simulink model "Simulink_ControllerARMAX_BlaneRev"  (R2020b)
settings: Solver=VariableStepAuto  StartTime=0.0  StopTime=2400  RelTol=1e-3
values from neighbouring files (symbols this model uses):
  A = [a2, a1, a0]    [Controller_ARMAX_BlaneRev.m]    (also in Controller_SS_BlaneRev.m; Controller_TF_BlaneRev.m = [a1, a0])
  B = [b2, b1, b0]    [Controller_ARMAX_BlaneRev.m]    (also in Controller_SS_BlaneRev.m; Controller_TF_BlaneRev.m = [b1, b0])
  b = double(sol.b)    [Controller_ARMAX_BlaneRev.m]    (also in Controller_SS_BlaneRev.m; Controller_TF_BlaneRev.m = double(sol))
  b_tun = 1    [Controller_ARMAX_BlaneRev.m]    (also in Controller_SS_BlaneRev.m = 0.04062; Controller_TF_BlaneRev.m = 0.008893)
  c = double(sol.c)    [Controller_ARMAX_BlaneRev.m]    (also in Controller_SS_BlaneRev.m)
  c0_Gc = (S0 + S1 + S2)/(1+r0)    [Controller_ARMAX_BlaneRev.m]    (also in Controller_SS_BlaneRev.m)
  c0_Gff = (T_S2 + T_S1 + T_S0)/(1+r0)    [Controller_ARMAX_BlaneRev.m]    (also in Controller_SS_BlaneRev.m)
  c_tun = 1    [Controller_ARMAX_BlaneRev.m]    (also in Controller_SS_BlaneRev.m = 0.0007977)
  D = double(sol.D)    [Controller_ARMAX_BlaneRev.m]    (also in Controller_SS_BlaneRev.m)
  D_tun = 109.2    [Controller_ARMAX_BlaneRev.m]    (also in Controller_SS_BlaneRev.m = 126.3)
  Gp = tf(sysARMAX)    [Controller_ARMAX_BlaneRev.m]    (also in Controller_SS_BlaneRev.m = tf(B, A, Ts2); Controller_TF_BlaneRev.m = tf(sysTF))
  Gp_cont = d2c(Gp_origin, 'zoh')    [Controller_ARMAX_BlaneRev.m]    (also in Controller_SS_BlaneRev.m; Controller_TF_BlaneRev.m = d2c(Gp, 'zoh'))
  I = double(sol.I)    [Controller_ARMAX_BlaneRev.m]    (also in Controller_SS_BlaneRev.m; Controller_TF_BlaneRev.m)
  I_tun = .06907    (= 0.06907)    [Controller_ARMAX_BlaneRev.m]    (also in Controller_SS_BlaneRev.m = 0.1006; Controller_TF_BlaneRev.m = 0.08704)
  N = double(sol.N)    [Controller_ARMAX_BlaneRev.m]    (also in Controller_SS_BlaneRev.m; systemIdentification_47414_Blane.m = 5; systemIdentification_48404_Blane.m = 5; systemIdentification_49404_Blane.m = 5)
  N_tun = .6217    (= 0.6217)    [Controller_ARMAX_BlaneRev.m]    (also in Controller_SS_BlaneRev.m = 0.5253)
  P = double(sol.P)    [Controller_ARMAX_BlaneRev.m]    (also in Controller_SS_BlaneRev.m; Controller_TF_BlaneRev.m)
  P_tun = 5.628    [Controller_ARMAX_BlaneRev.m]    (also in Controller_SS_BlaneRev.m = 7.185; Controller_TF_BlaneRev.m = 3.173)
  PD_den = [1, r0]    [Controller_ARMAX_BlaneRev.m]    (also in Controller_SS_BlaneRev.m)
  PD_SR_num = [d1_Gc, d0_Gc]    [Controller_ARMAX_BlaneRev.m]    (also in Controller_SS_BlaneRev.m)
  PD_TR_num = [d1_Gff, d0_Gff]    [Controller_ARMAX_BlaneRev.m]    (also in Controller_SS_BlaneRev.m)
  Ts = .4    (= 0.4)    [Controller_ARMAX_BlaneRev.m]    (also in Controller_SS_BlaneRev.m; Controller_TF_BlaneRev.m; systemIdentification_47414_Blane.m = 0.2; systemIdentification_48404_Blane.m = 1)
  Ts2 = .4    (= 0.4)    [Controller_ARMAX_BlaneRev.m]    (also in Controller_SS_BlaneRev.m; Controller_TF_BlaneRev.m)
  Ts3 = 1    [Controller_ARMAX_BlaneRev.m]    (also in Controller_SS_BlaneRev.m; Controller_TF_BlaneRev.m)
undefined symbols (not defined in the file or in its folder): DiscIntNeverNeededParam, K_ant
libraries: simulink_extras x8, pid_lib x2
settings Model: Creator=Blane Brinkley  LastModifiedBy=Blane Brinkley

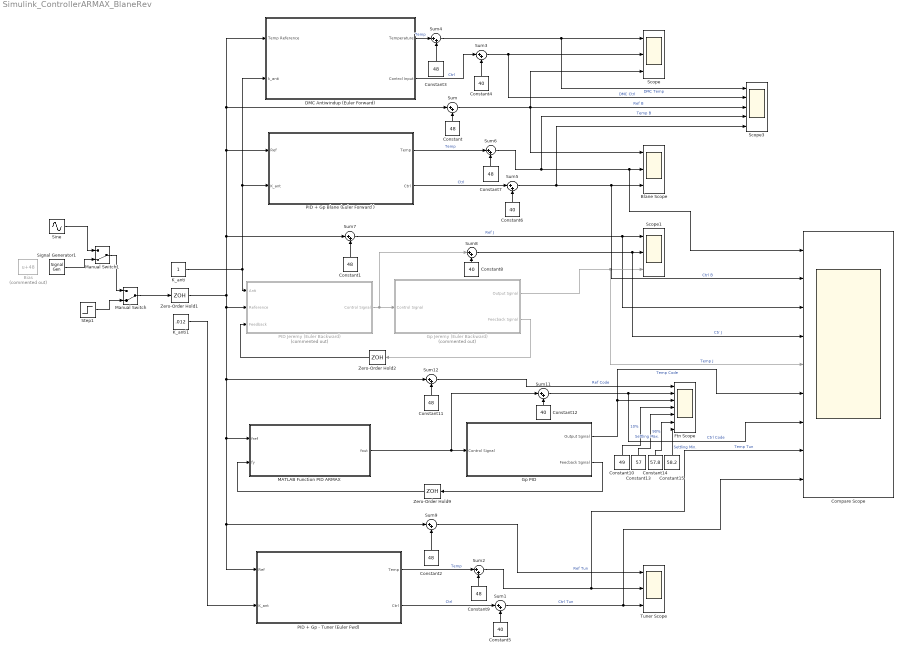
== system Simulink_ControllerARMAX_BlaneRev ==
  Bias : Bias  Commented=on  Bias=48
  Blane Scope : Scope  NumInputPorts=3
  Compare Scope : Scope  NumInputPorts=9
  Constant{,1..3,7,9,11} (7 alike) : Constant  Value=48
  Constant10 : Constant  Value=49
  Constant{4..6,8,12} (5 alike) : Constant  Value=40
  Constant13 : Constant  Value=57
  Constant14 : Constant  Value=57.8
  Constant15 : Constant  Value=58.2
  DMC Antiwindup (Euler Forward) : Subsystem
  Ftn Scope : Scope  NumInputPorts=7
  Gp Jeremy (Euler Backward) : Subsystem  Commented=on
  "Gp PID " : Subsystem
  K_anti : Constant
  K_anti1 : Constant  Value=.012  VectorParams1D=off
  MATLAB Function PID ARMAX : MATLAB Function  TreatAsAtomicUnit=on
  Manual Switch : ManualSwitch  CurrentSetting=0
  Manual Switch1 : ManualSwitch  CurrentSetting=0
  PID + Gp - Tuner (Euler Fwd) : Subsystem
  PID + Gp Blane (Euler Forward ) : Subsystem
  PID Jeremy (Euler Backward) : Subsystem  Commented=on
  Scope : Scope  NumInputPorts=3
  Scope1 : Scope  NumInputPorts=3
  Scope3 : Scope  NumInputPorts=5
  Signal Generator1 : SignalGenerator  WaveForm=square  Amplitude=20  Frequency=1/1200
  Sine : Sin  Amplitude=10  Frequency=1/1200*6.28  SampleTime=0
  Step1 : Step  Time=0  After=10  SampleTime=Ts
  Sum{,1..9,11..12} (12 alike) : Sum  Inputs=|++
  Tuner Scope : Scope  NumInputPorts=3
  Zero-Order Hold1 : ZeroOrderHold  SampleTime=Ts3
  Zero-Order Hold2 : ZeroOrderHold  SampleTime=Ts3
  Zero-Order Hold9 : ZeroOrderHold  SampleTime=Ts3
  wires:
  Signal Generator1/1 -> Manual Switch1/2
  Constant15/1 -> Ftn Scope/7  "Settling Min."
  Sine/1 -> Manual Switch1/1
  Manual Switch1/1 -> Manual Switch/1
  Constant14/1 -> Ftn Scope/6  "Settling Max."
  Step1/1 -> Manual Switch/2
  Zero-Order Hold2/1 -> PID Jeremy (Euler Backward)/3(Feedback)
  Constant2/1 -> Sum9/2
  Sum12/1 -> Ftn Scope/1  "Ref Code"
  Sum7/1 -> Compare Scope/3, Scope1/1  "Ref J"
  Constant3/1 -> Sum4/2
  Constant7/1 -> Sum6/2
  Constant4/1 -> Sum3/2
  PID Jeremy (Euler Backward)/1(Control Signal) -> Sum8/1, Gp Jeremy (Euler Backward)/1(Control Signal)
  Zero-Order Hold1/1 -> PID Jeremy (Euler Backward)/2(Reference), Sum12/1, PID + Gp - Tuner (Euler Fwd)/1(Ref), Sum9/1, MATLAB Function PID ARMAX/1(fref), DMC Antiwindup (Euler Forward)/1(Temp Reference), Sum/1, PID + Gp Blane (Euler Forward )/1(Ref), Sum7/1
  Sum/1 -> Scope3/3, Scope/3, Blane Scope/1  "Ref B"
  Sum4/1 -> Scope/1, Scope3/1  "DMC Temp"
  Constant/1 -> Sum/2
  DMC Antiwindup (Euler Forward)/1("Temperature ") -> Sum4/1  "Temp"
  Sum6/1 -> Scope3/4, Compare Scope/1, Blane Scope/2  "Temp B"
  PID + Gp Blane (Euler Forward )/1(Temp) -> Sum6/1  "Temp"
  Constant6/1 -> Sum5/2
  Constant1/1 -> Sum7/2
  Sum2/1 -> Compare Scope/8, Tuner Scope/2  "Temp Tun"
  Manual Switch/1 -> Zero-Order Hold1/1
  PID + Gp Blane (Euler Forward )/2(Ctrl) -> Sum5/1  "Ctrl"
  MATLAB Function PID ARMAX/1(fout) -> Sum11/1, "Gp PID "/1(Control Signal)
  "Gp PID "/1(Output Sginal) -> Compare Scope/6, Ftn Scope/3  "Temp Code"
  Gp Jeremy (Euler Backward)/1(Output Sginal) -> Compare Scope/5, Scope1/3  "Temp J"
  Sum5/1 -> Scope3/5, Compare Scope/2, Blane Scope/3  "Ctrl B"
  Sum8/1 -> Compare Scope/4, Scope1/2  "Ctr J"
  Constant12/1 -> Sum11/2
  DMC Antiwindup (Euler Forward)/2("Control Input ") -> Sum3/1  "Ctrl"
  Constant8/1 -> Sum8/2
  K_anti1/1 -> PID + Gp - Tuner (Euler Fwd)/2(K_ant)
  PID + Gp - Tuner (Euler Fwd)/2(Ctrl) -> Sum1/1  "Ctrl"
  Sum11/1 -> Compare Scope/7, Ftn Scope/2  "Ctrl Code"
  Sum1/1 -> Tuner Scope/3, Compare Scope/9  "Ctrl Tun"
  K_anti/1 -> PID Jeremy (Euler Backward)/1(Anti), DMC Antiwindup (Euler Forward)/2(k_anti), PID + Gp Blane (Euler Forward )/2(K_ant)
  "Gp PID "/2(Feecback Sginal) -> Zero-Order Hold9/1
  Constant9/1 -> Sum2/2
  Sum9/1 -> Tuner Scope/1  "Ref Tun"
  Constant5/1 -> Sum1/2
  Sum3/1 -> Scope/2, Scope3/2  "DMC Ctrl"
  Constant11/1 -> Sum12/2
  Gp Jeremy (Euler Backward)/2(Feecback Sginal) -> Zero-Order Hold2/1
  Zero-Order Hold9/1 -> MATLAB Function PID ARMAX/2(fy)
  Constant10/1 -> Ftn Scope/4  "10%"
  PID + Gp - Tuner (Euler Fwd)/1(Temp) -> Sum2/1  "Temp"
  Constant13/1 -> Ftn Scope/5  "90%"

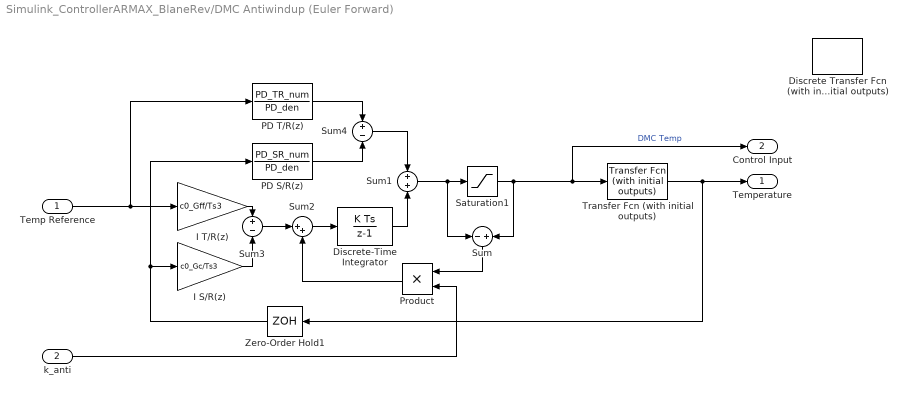
== system Simulink_ControllerARMAX_BlaneRev/DMC Antiwindup (Euler Forward) ==
  Temp Reference : Inport
  k_anti : Inport  Port=2
  Discrete Transfer Fcn (with initial outputs) : simulink_extras/Additional Discrete/Discrete Transfer Fcn (with initial outputs)  N=Gp.Numerator{1}  D=Gp.Denominator{1}  U0=[1]  Y0=0  TS=Ts
      settings: SourceProductBaseCode=SL
  Discrete-Time Integrator : DiscreteIntegrator  SampleTime=Ts3  ICPrevOutput=DiscIntNeverNeededParam  ICPrevScaledInput=DiscIntNeverNeededParam
  I S/R(z) : Gain  Gain=c0_Gc/Ts3
  I T/R(z) : Gain  Gain=c0_Gff/Ts3
  PD S/R(z) : DiscreteTransferFcn  Numerator=PD_SR_num  Denominator=PD_den  SampleTime=Ts3
  PD T/R(z) : DiscreteTransferFcn  Numerator=PD_TR_num  Denominator=PD_den  SampleTime=Ts3
  Product : Product
  Saturation1 : Saturate  UpperLimit=60  LowerLimit=-40
  Sum : Sum  Inputs=-+
  Sum1 : Sum
  Sum2 : Sum  Inputs=|++
  Sum3 : Sum  Inputs=+-
  Sum4 : Sum  Inputs=+-
  Transfer Fcn (with initial outputs) : simulink_extras/Additional Linear/Transfer Fcn (with initial outputs)  N=Gp_cont.Numerator{1}  D=Gp_cont.Denominator{1}  Y0=0  U0=0
  Zero-Order Hold1 : ZeroOrderHold  SampleTime=Ts3
  "Temperature " : Outport
  "Control Input " : Outport  Port=2
  wires:
  Sum3/1 -> Sum2/1
  I S/R(z)/1 -> Sum3/2
  Sum2/1 -> Discrete-Time Integrator/1
  I T/R(z)/1 -> Sum3/1
  Discrete-Time Integrator/1 -> Sum1/2
  Sum1/1 -> Sum/1, Saturation1/1
  Sum/1 -> Product/1
  Sum4/1 -> Sum1/1
  PD S/R(z)/1 -> Sum4/2
  PD T/R(z)/1 -> Sum4/1
  Product/1 -> Sum2/2
  Temp Reference/1 -> PD T/R(z)/1, I T/R(z)/1
  Transfer Fcn (with initial outputs)/1 -> Zero-Order Hold1/1, "Temperature "/1
  Zero-Order Hold1/1 -> I S/R(z)/1, PD S/R(z)/1
  Saturation1/1 -> Transfer Fcn (with initial outputs)/1, "Control Input "/1, Sum/2  "DMC Temp"
  k_anti/1 -> Product/2

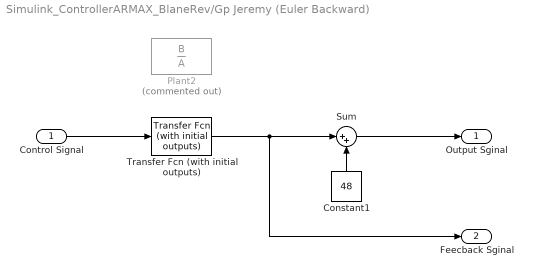
== system Simulink_ControllerARMAX_BlaneRev/Gp Jeremy (Euler Backward) ==
  Control Signal : Inport
  Constant1 : Constant  Value=48
  Plant2 : DiscreteTransferFcn  Commented=on  Numerator=B  Denominator=A  SampleTime=0.4
  Sum : Sum  Inputs=|++
  Transfer Fcn (with initial outputs) : simulink_extras/Additional Linear/Transfer Fcn (with initial outputs)  N=Gp_cont.Numerator{1}  D=Gp_cont.Denominator{1}  Y0=0  U0=0
  Output Sginal : Outport
  Feecback Sginal : Outport  Port=2
  wires:
  Transfer Fcn (with initial outputs)/1 -> Feecback Sginal/1, Sum/1
  Sum/1 -> Output Sginal/1
  Constant1/1 -> Sum/2
  Control Signal/1 -> Transfer Fcn (with initial outputs)/1

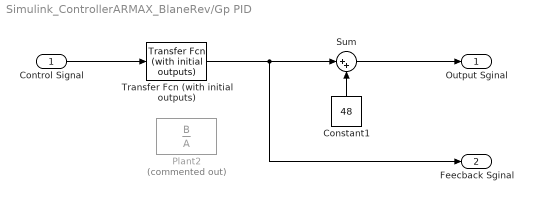
== system Simulink_ControllerARMAX_BlaneRev/Gp PID  ==
  Control Signal : Inport
  Constant1 : Constant  Value=48
  Plant2 : DiscreteTransferFcn  Commented=on  Numerator=B  Denominator=A  SampleTime=0.4
  Sum : Sum  Inputs=|++
  Transfer Fcn (with initial outputs) : simulink_extras/Additional Linear/Transfer Fcn (with initial outputs)  N=Gp_cont.Numerator{1}  D=Gp_cont.Denominator{1}  Y0=0  U0=0
  Output Sginal : Outport
  Feecback Sginal : Outport  Port=2
  wires:
  Transfer Fcn (with initial outputs)/1 -> Feecback Sginal/1, Sum/1
  Sum/1 -> Output Sginal/1
  Constant1/1 -> Sum/2
  Control Signal/1 -> Transfer Fcn (with initial outputs)/1

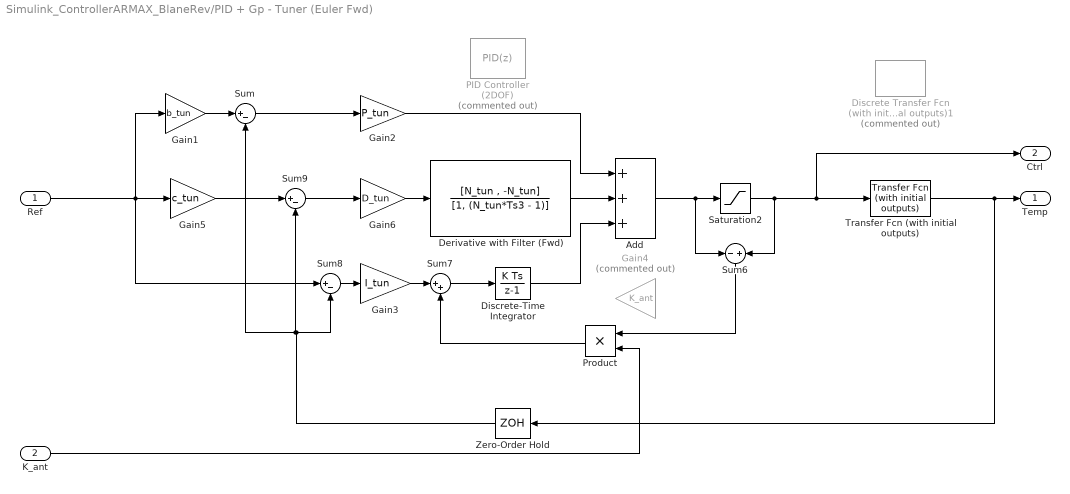
== system Simulink_ControllerARMAX_BlaneRev/PID + Gp - Tuner (Euler Fwd) ==
  Ref : Inport
  K_ant : Inport  Port=2
  Add : Sum  Inputs=+++
  Derivative with Filter (Fwd) : DiscreteTransferFcn  Numerator=[N_tun , -N_tun]  Denominator=[1, (N_tun*Ts3 - 1)]  SampleTime=Ts3
  Discrete Transfer Fcn (with initial outputs)1 : simulink_extras/Additional Discrete/Discrete Transfer Fcn (with initial outputs)  Commented=on  N=Gp.Numerator{1}  D=Gp.Denominator{1}  U0=[1]  Y0=0  TS=Ts
      settings: SourceProductBaseCode=SL
  Discrete-Time Integrator : DiscreteIntegrator  SampleTime=Ts3  ICPrevOutput=DiscIntNeverNeededParam  ICPrevScaledInput=DiscIntNeverNeededParam
  Gain1 : Gain  Gain=b_tun
  Gain2 : Gain  Gain=P_tun
  Gain3 : Gain  Gain=I_tun
  Gain4 : Gain  Commented=on  Gain=K_ant
  Gain5 : Gain  Gain=c_tun
  Gain6 : Gain  Gain=D_tun
  PID Controller (2DOF) : pid_lib/PID Controller (2DOF)  Commented=on  Controller=PID  Form=Parallel  TimeDomain=Discrete-time  UseExternalTs=off  SampleTime=-1  IntegratorMethod=Forward Euler  FilterMethod=Forward Euler  ControllerParametersSource=internal  P=1  I=1  D=0  UseFilter=on  N=100  b=1  c=1  TunerSelectOption=Transfer Function Based (PID Tuner App)  InitialConditionSource=internal  InitialConditionForIntegrator=0  InitialConditionForFilter=0  DifferentiatorICPrevScaledInput=0  ExternalReset=none  TrackingMode=off  Kt=1  LimitOutput=off  SatLimitsSource=internal  UpperSaturationLimit=inf  LowerSaturationLimit=-inf  LinearizeAsGain=on  AntiWindupMode=none  Kb=1  POutMin=[]  POutMax=[]  IOutMin=[]  IOutMax=[]  DOutMin=[]  DOutMax=[]  NOutMin=[]  NOutMax=[]  bOutMin=[]  bOutMax=[]  cOutMin=[]  cOutMax=[]  SumOutMin=[]  SumOutMax=[]  SaturationOutMin=[]  SaturationOutMax=[]  PParamMin=[]  PParamMax=[]  IParamMin=[]  IParamMax=[]  DParamMin=[]  DParamMax=[]  NParamMin=[]  NParamMax=[]  bParamMin=[]  bParamMax=[]  cParamMin=[]  cParamMax=[]  KbParamMin=[]  KbParamMax=[]  KtParamMin=[]  KtParamMax=[]  KbOutMin=[]  KbOutMax=[]  KtOutMin=[]  KtOutMax=[]  IntegratorOutMin=[]  IntegratorOutMax=[]  FilterOutMin=[]  FilterOutMax=[]  SumI1OutMin=[]  SumI1OutMax=[]  SumI2OutMin=[]  SumI2OutMax=[]  SumI3OutMin=[]  SumI3OutMax=[]  SumI4OutMin=[]  SumI4OutMax=[]  SumDOutMin=[]  SumDOutMax=[]  Sum1OutMin=[]  Sum1OutMax=[]  Sum2OutMin=[]  Sum2OutMax=[]  Sum3OutMin=[]  Sum3OutMax=[]  DifferentiatorOutMin=[]  DifferentiatorOutMax=[]  FilterDiffOutCoefMin=[]  FilterDiffOutCoefMax=[]  ReciprocalOutMin=[]  ReciprocalOutMax=[]  SumDenOutMin=[]  SumDenOutMax=[]  SumNumOutMin=[]  SumNumOutMax=[]  DivideOutMin=[]  DivideOutMax=[]  UdiffTsProdOutMin=[]  UdiffTsProdOutMax=[]  NTsProdOutMin=[]  NTsProdOutMax=[]  UintegralTsProdOutMin=[]  UintegralTsProdOutMax=[]  UngainTsProdOutMin=[]  UngainTsProdOutMax=[]  IntegratorContinuousStateAttributes=''  IntegratorStateMustResolveToSignalObject=off  IntegratorRTWStateStorageClass=Auto  FilterContinuousStateAttributes=''  FilterStateMustResolveToSignalObject=off  FilterRTWStateStorageClass=Auto  ParallelPVariant=InternalParameters  IdealPVariant=Disabled  IVariant=InternalParameters  DVariant=InternalParameters  bVariant=InternalParameters  cVariant=InternalParameters  IntegratorVariant=Discrete  SatVariant=Disabled  AWVariant=Passthrough  PCopyVariant=Disabled  TRVariant=Disabled  FdbkBlocksVariant=Forward  IdealPFdbkVariant=Disabled  SatFdbkVariant=Disabled  DerivativeFilterVariant=ForwardEulerFilter  NVariant=InternalParameters  NCopyVariant=Disabled  FilterICVariant=InternalICsFilter  IntegratorICVariant=InternalICs  ExternalResetVariant=Disabled  TRSumVariant=Passthrough  SumFdbkVariant=Disabled  SumVariant=Sum_PID  TsampFilterVariant=InternalTs  TsampNgainVariant=Passthrough  TsampIntegralVariant=Passthrough  ExternalSaturationOutDataTypeStr=Inherit: Same as second input
      settings: SourceProductBaseCode=SL
  Product : Product
  Saturation2 : Saturate  UpperLimit=60  LowerLimit=-40
  Sum : Sum  Inputs=|+-
  Sum6 : Sum  Inputs=-+
  Sum7 : Sum  Inputs=|++
  Sum8 : Sum  Inputs=|+-
  Sum9 : Sum  Inputs=|+-
  Transfer Fcn (with initial outputs) : simulink_extras/Additional Linear/Transfer Fcn (with initial outputs)  N=Gp_cont.Numerator{1}  D=Gp_cont.Denominator{1}  Y0=0  U0=0
  Zero-Order Hold : ZeroOrderHold  SampleTime=Ts3
  Temp : Outport
  Ctrl : Outport  Port=2
  wires:
  Gain1/1 -> Sum/1
  Sum/1 -> Gain2/1
  Sum8/1 -> Gain3/1
  Sum6/1 -> Product/1
  Add/1 -> Sum6/1, Saturation2/1
  Sum7/1 -> Discrete-Time Integrator/1
  Transfer Fcn (with initial outputs)/1 -> Zero-Order Hold/1, Temp/1
  Gain5/1 -> Sum9/1
  Sum9/1 -> Gain6/1
  Gain2/1 -> Add/1
  Gain6/1 -> Derivative with Filter (Fwd)/1
  Derivative with Filter (Fwd)/1 -> Add/2
  Product/1 -> Sum7/2
  Discrete-Time Integrator/1 -> Add/3
  Gain3/1 -> Sum7/1
  Saturation2/1 -> Sum6/2, Transfer Fcn (with initial outputs)/1, Ctrl/1
  Zero-Order Hold/1 -> Sum8/2, Sum9/2, Sum/2
  Ref/1 -> Sum8/1, Gain5/1, Gain1/1
  K_ant/1 -> Product/2

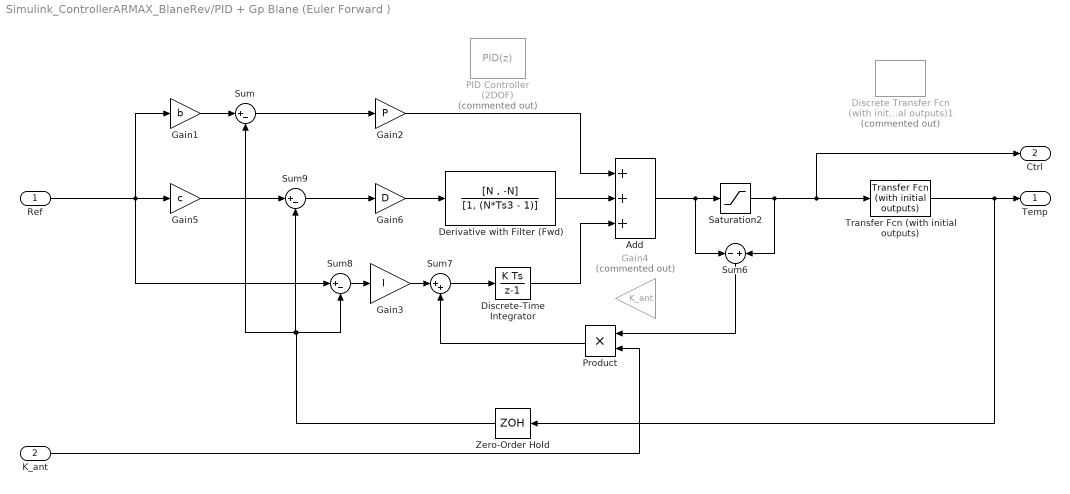
== system Simulink_ControllerARMAX_BlaneRev/PID + Gp Blane (Euler Forward ) ==
  Ref : Inport
  K_ant : Inport  Port=2
  Add : Sum  Inputs=+++
  Derivative with Filter (Fwd) : DiscreteTransferFcn  Numerator=[N , -N]  Denominator=[1, (N*Ts3 - 1)]  SampleTime=Ts3
  Discrete Transfer Fcn (with initial outputs)1 : simulink_extras/Additional Discrete/Discrete Transfer Fcn (with initial outputs)  Commented=on  N=Gp.Numerator{1}  D=Gp.Denominator{1}  U0=[1]  Y0=0  TS=Ts
      settings: SourceProductBaseCode=SL
  Discrete-Time Integrator : DiscreteIntegrator  SampleTime=Ts3  ICPrevOutput=DiscIntNeverNeededParam  ICPrevScaledInput=DiscIntNeverNeededParam
  Gain1 : Gain  Gain=b
  Gain2 : Gain  Gain=P
  Gain3 : Gain  Gain=I
  Gain4 : Gain  Commented=on  Gain=K_ant
  Gain5 : Gain  Gain=c
  Gain6 : Gain  Gain=D
  PID Controller (2DOF) : pid_lib/PID Controller (2DOF)  Commented=on  Controller=PID  Form=Parallel  TimeDomain=Discrete-time  UseExternalTs=off  SampleTime=-1  IntegratorMethod=Forward Euler  FilterMethod=Forward Euler  ControllerParametersSource=internal  P=1  I=1  D=0  UseFilter=on  N=100  b=1  c=1  TunerSelectOption=Transfer Function Based (PID Tuner App)  InitialConditionSource=internal  InitialConditionForIntegrator=0  InitialConditionForFilter=0  DifferentiatorICPrevScaledInput=0  ExternalReset=none  TrackingMode=off  Kt=1  LimitOutput=off  SatLimitsSource=internal  UpperSaturationLimit=inf  LowerSaturationLimit=-inf  LinearizeAsGain=on  AntiWindupMode=none  Kb=1  POutMin=[]  POutMax=[]  IOutMin=[]  IOutMax=[]  DOutMin=[]  DOutMax=[]  NOutMin=[]  NOutMax=[]  bOutMin=[]  bOutMax=[]  cOutMin=[]  cOutMax=[]  SumOutMin=[]  SumOutMax=[]  SaturationOutMin=[]  SaturationOutMax=[]  PParamMin=[]  PParamMax=[]  IParamMin=[]  IParamMax=[]  DParamMin=[]  DParamMax=[]  NParamMin=[]  NParamMax=[]  bParamMin=[]  bParamMax=[]  cParamMin=[]  cParamMax=[]  KbParamMin=[]  KbParamMax=[]  KtParamMin=[]  KtParamMax=[]  KbOutMin=[]  KbOutMax=[]  KtOutMin=[]  KtOutMax=[]  IntegratorOutMin=[]  IntegratorOutMax=[]  FilterOutMin=[]  FilterOutMax=[]  SumI1OutMin=[]  SumI1OutMax=[]  SumI2OutMin=[]  SumI2OutMax=[]  SumI3OutMin=[]  SumI3OutMax=[]  SumI4OutMin=[]  SumI4OutMax=[]  SumDOutMin=[]  SumDOutMax=[]  Sum1OutMin=[]  Sum1OutMax=[]  Sum2OutMin=[]  Sum2OutMax=[]  Sum3OutMin=[]  Sum3OutMax=[]  DifferentiatorOutMin=[]  DifferentiatorOutMax=[]  FilterDiffOutCoefMin=[]  FilterDiffOutCoefMax=[]  ReciprocalOutMin=[]  ReciprocalOutMax=[]  SumDenOutMin=[]  SumDenOutMax=[]  SumNumOutMin=[]  SumNumOutMax=[]  DivideOutMin=[]  DivideOutMax=[]  UdiffTsProdOutMin=[]  UdiffTsProdOutMax=[]  NTsProdOutMin=[]  NTsProdOutMax=[]  UintegralTsProdOutMin=[]  UintegralTsProdOutMax=[]  UngainTsProdOutMin=[]  UngainTsProdOutMax=[]  IntegratorContinuousStateAttributes=''  IntegratorStateMustResolveToSignalObject=off  IntegratorRTWStateStorageClass=Auto  FilterContinuousStateAttributes=''  FilterStateMustResolveToSignalObject=off  FilterRTWStateStorageClass=Auto  ParallelPVariant=InternalParameters  IdealPVariant=Disabled  IVariant=InternalParameters  DVariant=InternalParameters  bVariant=InternalParameters  cVariant=InternalParameters  IntegratorVariant=Discrete  SatVariant=Disabled  AWVariant=Passthrough  PCopyVariant=Disabled  TRVariant=Disabled  FdbkBlocksVariant=Forward  IdealPFdbkVariant=Disabled  SatFdbkVariant=Disabled  DerivativeFilterVariant=ForwardEulerFilter  NVariant=InternalParameters  NCopyVariant=Disabled  FilterICVariant=InternalICsFilter  IntegratorICVariant=InternalICs  ExternalResetVariant=Disabled  TRSumVariant=Passthrough  SumFdbkVariant=Disabled  SumVariant=Sum_PID  TsampFilterVariant=InternalTs  TsampNgainVariant=Passthrough  TsampIntegralVariant=Passthrough  ExternalSaturationOutDataTypeStr=Inherit: Same as second input
      settings: SourceProductBaseCode=SL
  Product : Product
  Saturation2 : Saturate  UpperLimit=60  LowerLimit=-40
  Sum : Sum  Inputs=|+-
  Sum6 : Sum  Inputs=-+
  Sum7 : Sum  Inputs=|++
  Sum8 : Sum  Inputs=|+-
  Sum9 : Sum  Inputs=|+-
  Transfer Fcn (with initial outputs) : simulink_extras/Additional Linear/Transfer Fcn (with initial outputs)  N=Gp_cont.Numerator{1}  D=Gp_cont.Denominator{1}  Y0=0  U0=0
  Zero-Order Hold : ZeroOrderHold  SampleTime=Ts3
  Temp : Outport
  Ctrl : Outport  Port=2
  wires:
  Gain1/1 -> Sum/1
  Sum/1 -> Gain2/1
  Sum8/1 -> Gain3/1
  Sum6/1 -> Product/1
  Add/1 -> Sum6/1, Saturation2/1
  Sum7/1 -> Discrete-Time Integrator/1
  Transfer Fcn (with initial outputs)/1 -> Zero-Order Hold/1, Temp/1
  Gain5/1 -> Sum9/1
  Sum9/1 -> Gain6/1
  Gain2/1 -> Add/1
  Gain6/1 -> Derivative with Filter (Fwd)/1
  Derivative with Filter (Fwd)/1 -> Add/2
  Product/1 -> Sum7/2
  Discrete-Time Integrator/1 -> Add/3
  Gain3/1 -> Sum7/1
  Saturation2/1 -> Sum6/2, Transfer Fcn (with initial outputs)/1, Ctrl/1
  Zero-Order Hold/1 -> Sum8/2, Sum9/2, Sum/2
  Ref/1 -> Sum8/1, Gain1/1, Gain5/1
  K_ant/1 -> Product/2

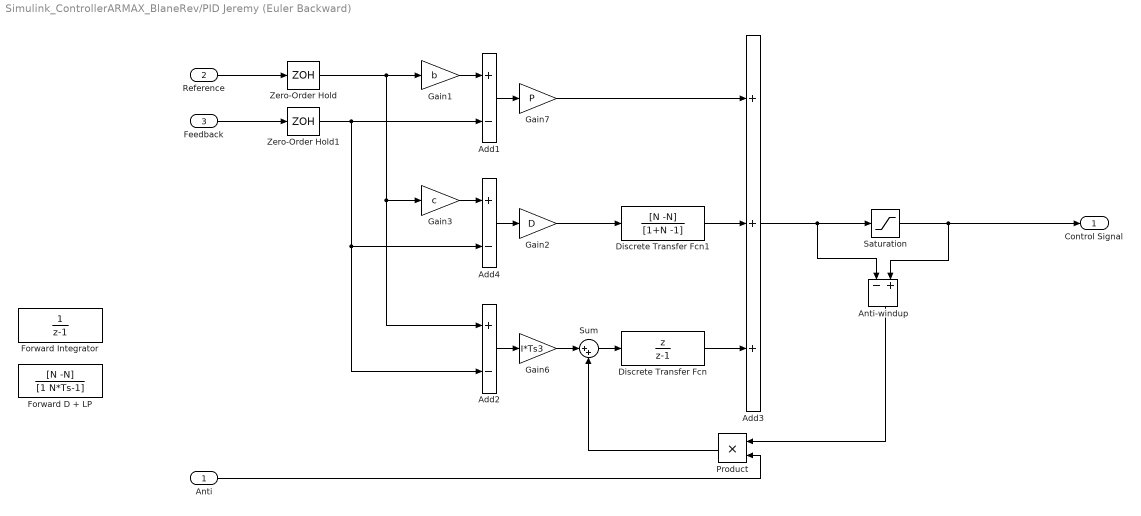
== system Simulink_ControllerARMAX_BlaneRev/PID Jeremy (Euler Backward) ==
  Anti : Inport
  Reference : Inport  Port=2
  Feedback : Inport  Port=3
  Add1 : Sum  Inputs=+-
  Add2 : Sum  Inputs=+-
  Add3 : Sum  Inputs=+++
  Add4 : Sum  Inputs=+-
  Anti-windup : Sum  Inputs=-+
  Discrete Transfer Fcn : DiscreteTransferFcn  Numerator=[1 0]  Denominator=[1 -1]  SampleTime=Ts2
  Discrete Transfer Fcn1 : DiscreteTransferFcn  Numerator=[N -N]  Denominator=[1+N -1]  SampleTime=Ts2
  Forward D + LP : DiscreteTransferFcn  Numerator=[N -N]  Denominator=[1 N*Ts-1]  SampleTime=Ts
  Forward Integrator : DiscreteTransferFcn  Denominator=[1 -1]  SampleTime=Ts
  Gain1 : Gain  Gain=b
  Gain2 : Gain  Gain=D
  Gain3 : Gain  Gain=c
  Gain6 : Gain  Gain=I*Ts3
  Gain7 : Gain  Gain=P
  Product : Product
  Saturation : Saturate  UpperLimit=60  LowerLimit=-40
  Sum : Sum  Inputs=|++
  Zero-Order Hold : ZeroOrderHold  SampleTime=Ts3
  Zero-Order Hold1 : ZeroOrderHold  SampleTime=Ts3
  Control Signal : Outport
  wires:
  Gain1/1 -> Add1/1
  Zero-Order Hold/1 -> Gain1/1, Gain3/1, Add2/1
  Reference/1 -> Zero-Order Hold/1
  Anti-windup/1 -> Product/1
  Product/1 -> Sum/2
  Add3/1 -> Saturation/1, Anti-windup/1
  Gain3/1 -> Add4/1
  Discrete Transfer Fcn1/1 -> Add3/2
  Add1/1 -> Gain7/1
  Gain7/1 -> Add3/1
  Add4/1 -> Gain2/1
  Gain2/1 -> Discrete Transfer Fcn1/1
  Add2/1 -> Gain6/1
  Discrete Transfer Fcn/1 -> Add3/3
  Sum/1 -> Discrete Transfer Fcn/1
  Gain6/1 -> Sum/1
  Feedback/1 -> Zero-Order Hold1/1
  Zero-Order Hold1/1 -> Add1/2, Add4/2, Add2/2
  Saturation/1 -> Control Signal/1, Anti-windup/2
  Anti/1 -> Product/2

== matlab function Simulink_ControllerARMAX_BlaneRev/MATLAB Function PID ARMAX ==
  data: fref input; fout output; fy input
function fout = fcn(fref, fy)
%%%%%%%%%%%%%%%%%%%%%%%%%%%%%%%%%%%%%%%%%%%%%%%%%%%%%%%
% PID + LP + PP for ARMAX
% Input : fref - reference signal
%         fy   - feedback signal
% Output: fout - control signal
%%%%%%%%%%%%%%%%%%%%%%%%%%%%%%%%%%%%%%%%%%%%%%%%%%%%%%%
% Variable Initialisation
persistent fD_prev fI_prev fIA_prev fDErr_prev fant;

% % Blane - SMALL ()
% Ts = 1;
% P = 8.1299;
% I = 0.1071;
% D = 109.7073;
% N = 0.1077;
% b = 0.8236;
% c = 0.6920;
% Kant = .045;

% Jeremy - SMALL ()
Ts = 1;
P = 2.987;
I = .03895;
D = 5.816;
N = .851;
b = 1;
c = 1;
Kant = .12;

% ----------------------------------------

% % Blane - LARGE (60.17 sec)
% Ts = 1;
% P = 57.5573;
% I = 1.5134;
% D = 923.3159;
% N = .5725;
% b = .1292;
% c = .0041;
% Kant = 1;

% % Jeremy - LARGE():
% Ts = 1;
% P = 5.628;
% I = .06907;
% D = 109.2;
% N = .6217;
% b = 1;
% c = 1;
% Kant = .012;

if isempty(fD_prev)
    fD_prev = 0;
    fI_prev = 0;
    fIA_prev = 0;
    fDErr_prev = 0;
    fant = 0;
    
end

fErr = fref - fy;
fDErr = fref*c - fy;

% P
fP = P*(b*fref - fy);
% D
fD = (D*N*(fDErr - fDErr_prev) + fD_prev)/(1+N*Ts);
% I
fI = fI_prev + fErr*I*Ts;
% Kant
fIA = fIA_prev + Kant*fant;

fsum = fP + fD + fI + fIA;

if fsum > 60
    fout = 60;
elseif fsum < (-40)
    fout = -40;
else
    fout = fsum;
end

% Update values
fDErr_prev = fDErr;
fD_prev = fD;
fI_prev = fI;
fIA_prev = fIA;
fant = fout - fsum;
end
